simulink model "gm_hybrid_lht"  (R2019b)
settings: Solver=FixedStepDiscrete  StartTime=0.0  StopTime=inf  FixedStep=1/120e6  RelTol=1e-3
undefined symbols (not defined in the file or in its folder): bt, height, nTheta, width
libraries: hdlsllib x672, simulink x614, hdlmdlgenlib x7, dspsrcs4 x1
(part 1 of 18)
settings Model: SimulationMode=accelerator  ExtModeTrigDuration=100  Creator=rgb11127  LastModifiedBy=rgb11127
settings DataIOCC: SaveOutput=off  SaveTime=off  ReturnWorkspaceOutputs=off  StateSaveName=tmp_raccel_xout  SignalLoggingName=tmp_raccel_logsout
settings OptimizationCC: BlockReduction=off  ConditionallyExecuteInputs=off  DefaultParameterBehavior=Inlined  EfficientMapNaN2IntZero=off
settings DebuggingCC: AlgebraicLoopMsg=error  InheritedTsInSrcMsg=none  SingleTaskRateTransMsg=error  ArithmeticOperatorsInVariantConditions=warning
settings HardwareCC: ProdBitPerPointer=32  ProdBitPerSizeT=32  ProdBitPerPtrDiffT=32  ProdLargestAtomicFloat=None  ProdIntDivRoundTo=Undefined  ProdEndianess=Unspecified  ProdWordSize=32  ProdHWDeviceType=ASIC/FPGA->ASIC/FPGA  TargetBitPerPointer=64  TargetBitPerSizeT=64  TargetBitPerPtrDiffT=64  TargetLongLongMode=on  TargetIntDivRoundTo=Zero  TargetEndianess=LittleEndian  TargetWordSize=64  TargetHWDeviceType=Custom Processor->MATLAB Host Computer  ProdEqTarget=off
settings SFSimCC: CustomCodeUndefinedFunction=UseInterfaceOnly
settings RTWCC: SystemTargetFile=raccel.tlc  TemplateMakefile=raccel_default_tmf  RTWVerbose=off  RTWUseSimCustomCode=on
settings CodeAppCC: GenerateComments=off  MaxIdLength=128
settings RaccelTargetCC: GeneratePreprocessorConditionals=Use local settings  MultiInstanceERTCode=off  PreserveStateflowLocalDataDimensions=off  ExtModeMexArgs='', 0, 56287  ENABLE_SLEXEC_SSBRIDGE=1  RTWCAPIParams=on

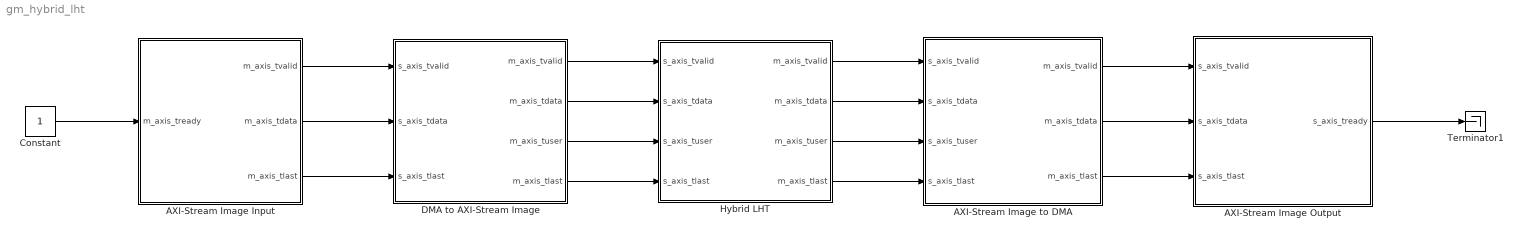
== system gm_hybrid_lht ==
  AXI-Stream Image Input : Subsystem  mask{image=bt.inputImage, clk=1/120e6}
      mask prompts: image "Input Image:"; clk "Clock Rate:"
      mask init:
      | [height, width] = size(image);
      mask DialogControl DescGroupVar Prompt: AXI-Stream Image Input
      mask DialogControl DescTextVar Prompt: This block simulates an AXI-Stream image input for interfacing to a hardware accelerator or IP Core.
      mask DialogControl ParameterGroupVar Prompt: Main
  AXI-Stream Image Output : Subsystem  mask{height=bt.nRho, width=bt.nTheta, clk=1/120e6, d=0}
      mask prompts: height "Image Height:"; width "Image Width:"; clk "Clock Rate:"; d "Frame Capture Number"
      mask DialogControl DescGroupVar Prompt: AXI-Stream Image Output
      mask DialogControl DescTextVar Prompt: Image output using the AXI-Stream interface. Simulates an AXI DMA write channel.
      mask DialogControl ParameterGroupVar Prompt: Main
  AXI-Stream Image to DMA : Subsystem  mask{height=bt.nRho, width=bt.nTheta}
      mask prompts: height "Image Height"; width "Image Width"
      mask DialogControl DescGroupVar Prompt: AXI-Stream Image to DMA
      mask DialogControl DescTextVar Prompt: Converts from the AXI-Stream video standard to AXI-Stream DMA packet.
      mask DialogControl Container2 Prompt: Main
  Constant : Constant  OutDataTypeStr=boolean  SampleTime=-1
  DMA to AXI-Stream Image : Subsystem  mask{height=bt.height, width=bt.width}
      mask prompts: height "Image Height:"; width "Image Width:"
      mask DialogControl DescGroupVar Prompt: DMA to AXI-Stream Image
      mask DialogControl DescTextVar Prompt: Converts an DMA AXI-Stream packet to the AXI-Stream video standard.
      mask DialogControl Container2 Prompt: Main
  Hybrid LHT : Subsystem
  Terminator1 : Terminator
  wires:
  Constant/1 -> AXI-Stream Image Input/1(m_axis_tready)
  AXI-Stream Image Input/1(m_axis_tvalid) -> DMA to AXI-Stream Image/1(s_axis_tvalid)
  AXI-Stream Image Input/2(m_axis_tdata) -> DMA to AXI-Stream Image/2(s_axis_tdata)
  AXI-Stream Image Input/3(m_axis_tlast) -> DMA to AXI-Stream Image/3(s_axis_tlast)
  DMA to AXI-Stream Image/1(m_axis_tvalid) -> Hybrid LHT/1(s_axis_tvalid)
  DMA to AXI-Stream Image/2(m_axis_tdata) -> Hybrid LHT/2(s_axis_tdata)
  DMA to AXI-Stream Image/3(m_axis_tuser) -> Hybrid LHT/3(s_axis_tuser)
  DMA to AXI-Stream Image/4(m_axis_tlast) -> Hybrid LHT/4(s_axis_tlast)
  AXI-Stream Image Output/1(s_axis_tready) -> Terminator1/1
  AXI-Stream Image to DMA/3(m_axis_tlast) -> AXI-Stream Image Output/3(s_axis_tlast)
  AXI-Stream Image to DMA/2(m_axis_tdata) -> AXI-Stream Image Output/2(s_axis_tdata)
  AXI-Stream Image to DMA/1(m_axis_tvalid) -> AXI-Stream Image Output/1(s_axis_tvalid)
  Hybrid LHT/4(m_axis_tlast) -> AXI-Stream Image to DMA/4(s_axis_tlast)
  Hybrid LHT/3(m_axis_tuser) -> AXI-Stream Image to DMA/3(s_axis_tuser)
  Hybrid LHT/2(m_axis_tdata) -> AXI-Stream Image to DMA/2(s_axis_tdata)
  Hybrid LHT/1(m_axis_tvalid) -> AXI-Stream Image to DMA/1(s_axis_tvalid)

== system gm_hybrid_lht/AXI-Stream Image Input ==
  m_axis_tready : Inport
  Compare To Constant : simulink/Logic and Bit Operations/Compare To Constant  relop===  const=height*width-1  OutDataTypeStr=boolean
  Data Type Conversion : DataTypeConversion  OutDataTypeStr=fixdt(0, ceil(log2(max(max(double(image))))), 0)
  HDL Counter : hdlsllib/Sources/HDL Counter  CountType=Count limited  CountInit=0  CountStep=1  CountMax=width*height-1  CountFromType=Initial value  CountFrom=0  CountResetPort=off  CountLoadPort=off  CountEnbPort=on  CountDirPort=off  CountDataType=Unsigned  CountWordLen=ceil(log2(width*height))  CountFracLen=0  CountSampTime=1
      settings: SourceProductName=Simulink
  Master AXI-Stream FIFO : Subsystem  mask{depth=32}
      mask prompts: depth "FIFO Depth:"
      mask DialogControl DescGroupVar Prompt: Master AXI-Stream FIFO
      mask DialogControl DescTextVar Prompt: A custom AXI-Stream FIFO for interfacing to write channel AXI DMAs.
      mask DialogControl ParameterGroupVar Prompt: Main
  Synchronous Image Source : Subsystem
  m_axis_tvalid : Outport
  m_axis_tdata : Outport  Port=2
  m_axis_tlast : Outport  Port=3
  wires:
  Data Type Conversion/1 -> Master AXI-Stream FIFO/2(s_axis_tdata)
  Master AXI-Stream FIFO/2(m_axis_tdata) -> m_axis_tdata/1
  Master AXI-Stream FIFO/3(m_axis_tlast) -> m_axis_tlast/1
  m_axis_tready/1 -> Master AXI-Stream FIFO/4(m_axis_tready)
  Master AXI-Stream FIFO/4(s_axis_tready) -> HDL Counter/1, Master AXI-Stream FIFO/1(s_axis_tvalid), Synchronous Image Source/Enable
  Compare To Constant/1 -> Master AXI-Stream FIFO/3(s_axis_tlast)
  Master AXI-Stream FIFO/1(m_axis_tvalid) -> m_axis_tvalid/1
  HDL Counter/1 -> Compare To Constant/1
  Synchronous Image Source/1(Pixel) -> Data Type Conversion/1

== system gm_hybrid_lht/AXI-Stream Image Output ==
  s_axis_tvalid : Inport
  s_axis_tdata : Inport  Port=2
  s_axis_tlast : Inport  Port=3
  AND1 : Logic  IconShape=distinctive  AllPortsSameDT=off  OutDataTypeStr=boolean
  Compare To Constant4 : simulink/Logic and Bit Operations/Compare To Constant  relop===  const=(height)*width-1  OutDataTypeStr=boolean
  Constant : Constant  OutDataTypeStr=boolean  SampleTime=-1
  Delay2 : Delay  DelayLength=d  ShowEnablePort=on
      settings: InputPortMap=u0,e6
  Pixel to Workspace : Subsystem
  Stop Simulation1 : Stop
  Terminator : Terminator
  Total Samples Counter : hdlsllib/Sources/HDL Counter  CountType=Count limited  CountInit=0  CountStep=1  CountMax=(height)*width-1  CountFromType=Initial value  CountFrom=0  CountResetPort=off  CountLoadPort=off  CountEnbPort=on  CountDirPort=off  CountDataType=Unsigned  CountWordLen=ceil(log2((height)*width+1))  CountFracLen=0  CountSampTime=1
      settings: SourceProductName=Simulink
  s_axis_tready : Outport  VectorParamsAs1DForOutWhenUnconnected=off
  wires:
  Constant/1 -> s_axis_tready/1, AND1/2
  s_axis_tlast/1 -> Terminator/1
  Delay2/1 -> Stop Simulation1/1
  Compare To Constant4/1 -> Delay2/1, Delay2/2
  Total Samples Counter/1 -> Compare To Constant4/1
  AND1/1 -> Pixel to Workspace/Enable, Total Samples Counter/1
  s_axis_tvalid/1 -> AND1/1
  s_axis_tdata/1 -> Pixel to Workspace/1(Pixel In)

== system gm_hybrid_lht/AXI-Stream Image to DMA ==
  s_axis_tvalid : Inport
  s_axis_tdata : Inport  Port=2
  s_axis_tuser : Inport  Port=3
  s_axis_tlast : Inport  Port=4
  AND : Logic  IconShape=distinctive  AllPortsSameDT=off  OutDataTypeStr=boolean
  Compare To Constant : simulink/Logic and Bit Operations/Compare To Constant  relop===  const=height*width-1  OutDataTypeStr=boolean
  Data Type Conversion : DataTypeConversion  OutDataTypeStr=uint32
  Output Counter : hdlsllib/Sources/HDL Counter  CountType=Count limited  CountInit=0  CountStep=1  CountMax=height*width-1  CountFromType=Initial value  CountFrom=0  CountResetPort=off  CountLoadPort=off  CountEnbPort=on  CountDirPort=off  CountDataType=Unsigned  CountWordLen=ceil(log2(height*width))  CountFracLen=0  CountSampTime=1
      settings: SourceProductName=Simulink
  Terminator : Terminator
  Terminator1 : Terminator
  m_axis_tvalid : Outport
  m_axis_tdata : Outport  Port=2
  m_axis_tlast : Outport  Port=3
  wires:
  Data Type Conversion/1 -> m_axis_tdata/1
  s_axis_tdata/1 -> Data Type Conversion/1
  s_axis_tvalid/1 -> AND/2, m_axis_tvalid/1, Output Counter/1
  s_axis_tlast/1 -> Terminator/1
  s_axis_tuser/1 -> Terminator1/1
  Output Counter/1 -> Compare To Constant/1
  Compare To Constant/1 -> AND/1
  AND/1 -> m_axis_tlast/1

== system gm_hybrid_lht/DMA to AXI-Stream Image ==
  s_axis_tvalid : Inport
  s_axis_tdata : Inport  Port=2
  s_axis_tlast : Inport  Port=3
  AND : Logic  IconShape=distinctive  AllPortsSameDT=off  OutDataTypeStr=boolean
  AND1 : Logic  IconShape=distinctive  AllPortsSameDT=off  OutDataTypeStr=boolean
  AND2 : Logic  IconShape=distinctive  AllPortsSameDT=off  OutDataTypeStr=boolean
  Compare To Constant : simulink/Logic and Bit Operations/Compare To Constant  relop===  const=width-1  OutDataTypeStr=boolean
  Compare To Zero : simulink/Logic and Bit Operations/Compare To Zero  relop===  OutDataTypeStr=boolean
  Compare To Zero1 : simulink/Logic and Bit Operations/Compare To Zero  relop===  OutDataTypeStr=boolean
  Terminator : Terminator
  X Counter : hdlsllib/Sources/HDL Counter  CountType=Count limited  CountInit=0  CountStep=1  CountMax=width-1  CountFromType=Initial value  CountFrom=0  CountResetPort=off  CountLoadPort=off  CountEnbPort=on  CountDirPort=off  CountDataType=Unsigned  CountWordLen=ceil(log2(width))  CountFracLen=0  CountSampTime=1
      settings: SourceProductName=Simulink
  Y Counter : hdlsllib/Sources/HDL Counter  CountType=Count limited  CountInit=0  CountStep=1  CountMax=height-1  CountFromType=Initial value  CountFrom=0  CountResetPort=off  CountLoadPort=off  CountEnbPort=on  CountDirPort=off  CountDataType=Unsigned  CountWordLen=ceil(log2(height))  CountFracLen=0  CountSampTime=1
      settings: SourceProductName=Simulink
  m_axis_tvalid : Outport
  m_axis_tdata : Outport  Port=2
  m_axis_tuser : Outport  Port=3
  m_axis_tlast : Outport  Port=4
  wires:
  AND2/1 -> m_axis_tlast/1
  Compare To Constant/1 -> Y Counter/1, AND2/2
  AND1/1 -> m_axis_tuser/1
  AND/1 -> AND1/2
  s_axis_tlast/1 -> Terminator/1
  Compare To Zero/1 -> AND/2
  Compare To Zero1/1 -> AND/1
  Y Counter/1 -> Compare To Zero/1
  X Counter/1 -> Compare To Constant/1, Compare To Zero1/1
  s_axis_tvalid/1 -> m_axis_tvalid/1, AND1/1, AND2/1, X Counter/1
  s_axis_tdata/1 -> m_axis_tdata/1

== system gm_hybrid_lht/Hybrid LHT ==
  s_axis_tvalid : Inport  OutDataTypeStr=boolean  PortDimensions=1  SampleTime=8.33333333333333e-09
  s_axis_tdata : Inport  Port=2  OutDataTypeStr=fixdt(0, 9, 0)  PortDimensions=1  SampleTime=8.33333333333333e-09
  s_axis_tuser : Inport  Port=3  OutDataTypeStr=boolean  PortDimensions=1  SampleTime=8.33333333333333e-09
  s_axis_tlast : Inport  Port=4  OutDataTypeStr=boolean  PortDimensions=1  SampleTime=8.33333333333333e-09
  Hybrid LHT Accumulator : Subsystem  mask{height=double(1080), width=double(1920), theta=reshape(double([0 1 2 3 4 5 6 7 8 9 10 11 12 13 14 15 16 17 18 19 20 21 22 23 24 25 26 27 28 29 30 31 32 33 34 35 36 37 38 39 40 41 42 43 44 45 46 47 48 49 50 51 52 53 54 55 56 57 58 59 60 61 62 63 64 65 66 67 68 69 70 71 72 73 74 75 76 77 78 79 80 81 82 83 84 85 86 87 88 89 90 91 92 93 94 95 96 97 98 99 100 101 102 103 104 105 106 107 108 109 110 111 112 113 114 115 116 117 118 119 120 121 122 123 124 125 126 127 128 129 130 131 132 133 134 135 136 137 138 139 140 141 142 143 144 145 146 147 148 149 150 151 152 153 154 155 156 157 158 159 160 161 162 163 164 165 166 167 168 169 170 171 172 173 174 175 176 177 178 179]).', [1  180])}
      mask prompts: height "Image Height:"; width "Image Width:"; theta "Orientations:"
      mask init:
      | maxRho = ceil(sqrt((height/2)^2+(width/2)^2));
      | nRho = maxRho*2;
      | [~, nTheta] = size(theta);
      | 
      | voteWL = ceil(log2(2*maxRho));
  Hybrid LHT Kernel : Subsystem  mask{height=double(1080), width=double(1920), theta=reshape(double([0 1 2 3 4 5 6 7 8 9 10 11 12 13 14 15 16 17 18 19 20 21 22 23 24 25 26 27 28 29 30 31 32 33 34 35 36 37 38 39 40 41 42 43 44 45 46 47 48 49 50 51 52 53 54 55 56 57 58 59 60 61 62 63 64 65 66 67 68 69 70 71 72 73 74 75 76 77 78 79 80 81 82 83 84 85 86 87 88 89 90 91 92 93 94 95 96 97 98 99 100 101 102 103 104 105 106 107 108 109 110 111 112 113 114 115 116 117 118 119 120 121 122 123 124 125 126 127 128 129 130 131 132 133 134 135 136 137 138 139 140 141 142 143 144 145 146 147 148 149 150 151 152 153 154 155 156 157 158 159 160 161 162 163 164 165 166 167 168 169 170 171 172 173 174 175 176 177 178 179]).', [1  180])}
      mask prompts: height "Image Height:"; width "Image Width:"; theta "Orientations:"
      mask init:
      | % Get number of orientations to operate across
      | [~, nTheta] = size(theta);
      | 
      | % Get discretisation step of theta
      | if nTheta > 1
      |     dTheta = theta(end) - theta(end-1);
      | else
      |     dTheta = 1;
      | end
      | 
      | % Get the maximum magnitude of displacement
      | maxRho = ceil(sqrt((height/2)^2+(width/2)^2));
      | 
      | % Get the number of bits required to vote correctly
      | voteWL = ceil(log2(maxRho*2));
      | 
      | % Get the number of division possible
      | if nTheta < floor(36/voteWL)
      |     L = nTheta;
      | else
      |     L = floor(36/voteWL);
      | end
      | 
      | % Set lambda, the number of orientations to operate across per gradient
      | % orientation given
      | lambda = floor(nTheta/(2*L));
      | 
      | % Determine if the number of orientations is odd. This will prevent over
      | % use of the parameter space.
      | if lambda == 0
      |     subflag = 0;
      | else
      |     subflag = ~mod(nTheta/(L), 2);
      | end
      | 
      | % Get the limits so that we can determine the number of bits to shift
      | % the votes
      | U = floor(nTheta/L):floor(nTheta/L):nTheta;
      | D = 0:floor(nTheta/L):nTheta-1;
  delayMatch : Delay  DelayLength=double(2)  InitialCondition=0  SampleTime=8.33333333333333e-09
  delayMatch1 : Delay  DelayLength=double(2)  InitialCondition=0  SampleTime=8.33333333333333e-09
  m_axis_tvalid : Outport
  m_axis_tdata : Outport  Port=2
  m_axis_tuser : Outport  Port=3
  m_axis_tlast : Outport  Port=4
  wires:
  s_axis_tvalid/1 -> Hybrid LHT Kernel/1(s_axis_tvalid)
  s_axis_tdata/1 -> Hybrid LHT Kernel/2(s_axis_tdata)
  s_axis_tuser/1 -> Hybrid LHT Kernel/3(s_axis_tuser)
  s_axis_tlast/1 -> Hybrid LHT Kernel/4(s_axis_tlast)
  delayMatch/1 -> m_axis_tvalid/1
  Hybrid LHT Accumulator/2(m_axis_tdata) -> m_axis_tdata/1
  Hybrid LHT Accumulator/3(m_axis_tuser) -> m_axis_tuser/1
  delayMatch1/1 -> m_axis_tlast/1
  Hybrid LHT Kernel/1(m_axis_tvalid) -> Hybrid LHT Accumulator/1(s_axis_tvalid)
  Hybrid LHT Kernel/2(m_axis_tuser) -> Hybrid LHT Accumulator/2(s_axis_tuser)
  Hybrid LHT Kernel/3(m_axis_tlast) -> Hybrid LHT Accumulator/3(s_axis_tlast)
  Hybrid LHT Kernel/4(hough_param) -> Hybrid LHT Accumulator/4(hough_param)
  Hybrid LHT Kernel/5(edge) -> Hybrid LHT Accumulator/5(edge)
  Hybrid LHT Kernel/6(shift) -> Hybrid LHT Accumulator/6(shift)
  Hybrid LHT Accumulator/1(m_axis_tvalid) -> delayMatch/1
  Hybrid LHT Accumulator/4(m_axis_tlast) -> delayMatch1/1

== system gm_hybrid_lht/AXI-Stream Image Input/Master AXI-Stream FIFO ==
  s_axis_tvalid : Inport
  s_axis_tdata : Inport  Port=2
  s_axis_tlast : Inport  Port=3
  m_axis_tready : Inport  Port=4
  AND : Logic  IconShape=distinctive  AllPortsSameDT=off  OutDataTypeStr=boolean
  "Compare To Constant " : simulink/Logic and Bit Operations/Compare To Constant  relop=>=  const=floor(depth/2)  OutDataTypeStr=boolean
  Delay : Delay  DelayLength=1
  HDL FIFO TDATA : hdlsllib/HDL RAMs/HDL FIFO  fifo_size=depth  mode=Classic  ratio=1  push_msg=Error  pop_msg=Error  show_empty=on  show_full=off  show_num=on  LabelModeActiveChoice_Mode=Classic
      settings: SourceProductName=Simulink  SourceProductBaseCode=SL
  HDL FIFO TLAST : hdlsllib/HDL RAMs/HDL FIFO  fifo_size=depth  mode=Classic  ratio=1  push_msg=Error  pop_msg=Error  show_empty=off  show_full=off  show_num=off  LabelModeActiveChoice_Mode=Classic
      settings: SourceProductName=Simulink  SourceProductBaseCode=SL
  NOT : Logic  Operator=NOT  IconShape=distinctive  AllPortsSameDT=off  OutDataTypeStr=boolean
  NOT1 : Logic  Operator=NOT  IconShape=distinctive  AllPortsSameDT=off  OutDataTypeStr=boolean
  m_axis_tvalid : Outport  VectorParamsAs1DForOutWhenUnconnected=off
  m_axis_tdata : Outport  Port=2  VectorParamsAs1DForOutWhenUnconnected=off
  m_axis_tlast : Outport  Port=3  VectorParamsAs1DForOutWhenUnconnected=off
  s_axis_tready : Outport  Port=4
  wires:
  Delay/1 -> m_axis_tvalid/1
  s_axis_tvalid/1 -> HDL FIFO TDATA/2, HDL FIFO TLAST/2
  s_axis_tdata/1 -> HDL FIFO TDATA/1
  s_axis_tlast/1 -> HDL FIFO TLAST/1
  "Compare To Constant "/1 -> NOT1/1
  NOT1/1 -> s_axis_tready/1
  HDL FIFO TDATA/3 -> "Compare To Constant "/1
  m_axis_tready/1 -> AND/1
  NOT/1 -> AND/2, Delay/1
  AND/1 -> HDL FIFO TDATA/3, HDL FIFO TLAST/3
  HDL FIFO TDATA/2 -> NOT/1
  HDL FIFO TLAST/1 -> m_axis_tlast/1
  HDL FIFO TDATA/1 -> m_axis_tdata/1

== system gm_hybrid_lht/AXI-Stream Image Input/Synchronous Image Source ==
  Enable : EnablePort
  Signal From Workspace : dspsrcs4/Signal From Workspace  X=reshape((double(image))', [height*width, 1])  Ts=clk  nsamps=1  OutputAfterFinalValue=Cyclic repetition  ignoreOrWarnInputAndFrameLengths=off  OutputFrames=off
  Pixel : Outport
  wires:
  Signal From Workspace/1 -> Pixel/1

== system gm_hybrid_lht/AXI-Stream Image Output/Pixel to Workspace ==
  Pixel In : Inport
  Enable : EnablePort
  To Workspace : ToWorkspace  VariableName=simout  SampleTime=-1
      settings: MaxDataPoints=height*width  Save2DSignal=2-D array (concatenate along first dimension)
  wires:
  Pixel In/1 -> To Workspace/1

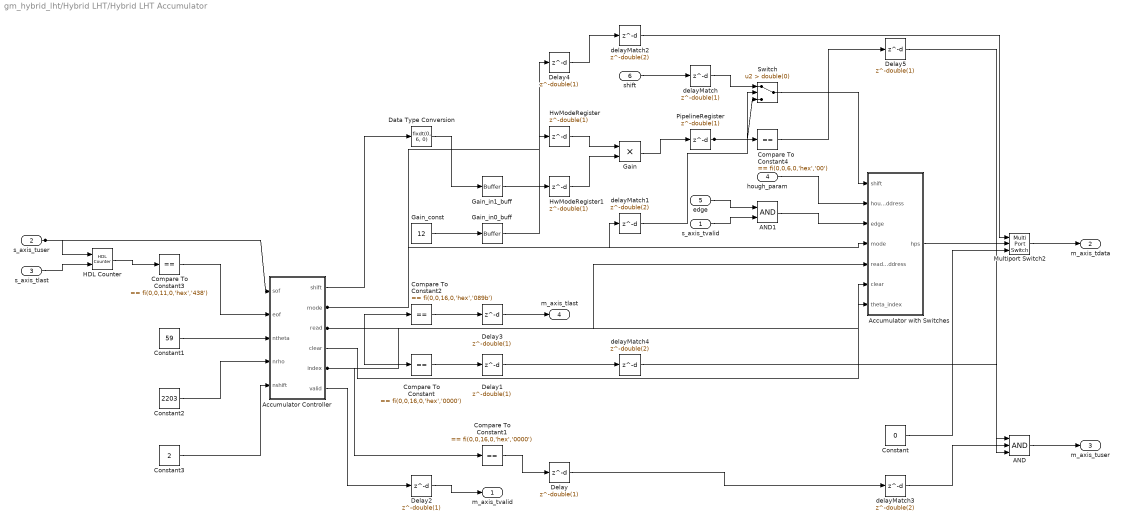
== system gm_hybrid_lht/Hybrid LHT/Hybrid LHT Accumulator ==
  s_axis_tvalid : Inport  OutDataTypeStr=boolean  PortDimensions=1  SampleTime=8.33333333333333e-09
  s_axis_tuser : Inport  Port=2  OutDataTypeStr=boolean  PortDimensions=1  SampleTime=8.33333333333333e-09
  s_axis_tlast : Inport  Port=3  OutDataTypeStr=boolean  PortDimensions=1  SampleTime=8.33333333333333e-09
  hough_param : Inport  Port=4  OutDataTypeStr=fixdt(0, 12, 0)  PortDimensions=[1 60]  SampleTime=8.33333333333333e-09
  edge : Inport  Port=5  OutDataTypeStr=fixdt(0, 1, 0)  PortDimensions=1  SampleTime=8.33333333333333e-09
  shift : Inport  Port=6  OutDataTypeStr=fixdt(0, 6, 0)  PortDimensions=[1 60]  SampleTime=8.33333333333333e-09
  AND : Logic  Inputs=3  AllPortsSameDT=off  OutDataTypeStr=boolean  SampleTime=8.33333333333333e-09
  AND1 : Logic  AllPortsSameDT=off  OutDataTypeStr=boolean  SampleTime=8.33333333333333e-09
  Accumulator Controller : Subsystem
  Accumulator with Switches : Subsystem
  Compare To Constant : simulink/Logic and Bit Operations/Compare To Constant  relop===  const=fi(0,0,16,0,'hex','0000')  OutDataTypeStr=boolean
  Compare To Constant1 : simulink/Logic and Bit Operations/Compare To Constant  relop===  const=fi(0,0,16,0,'hex','0000')  OutDataTypeStr=boolean
  Compare To Constant2 : simulink/Logic and Bit Operations/Compare To Constant  relop===  const=fi(0,0,16,0,'hex','089b')  OutDataTypeStr=boolean
  Compare To Constant3 : simulink/Logic and Bit Operations/Compare To Constant  relop===  const=fi(0,0,11,0,'hex','438')  OutDataTypeStr=boolean
  Compare To Constant4 : simulink/Logic and Bit Operations/Compare To Constant  relop===  const=fi(0,0,6,0,'hex','00')  OutDataTypeStr=boolean
  Constant : Constant  Value=0  OutDataTypeStr=fixdt(0, 12, 0)  SampleTime=-1
  Constant1 : Constant  Value=59  OutDataTypeStr=uint16  SampleTime=-1
  Constant2 : Constant  Value=2203  OutDataTypeStr=uint16  SampleTime=-1
  Constant3 : Constant  Value=2  OutDataTypeStr=fixdt(0, 3, 0)  SampleTime=-1
  Data Type Conversion : DataTypeConversion  OutDataTypeStr=fixdt(0, 6, 0)  SampleTime=8.33333333333333e-09
  Delay{,1..5} (6 alike) : Delay  DelayLength=double(1)  InitialCondition=0  SampleTime=8.33333333333333e-09
  Gain : Product  Inputs=**  OutDataTypeStr=fixdt(0, 6, 0)  SampleTime=8.33333333333333e-09
  Gain_const : Constant  Value=12  OutDataTypeStr=fixdt(0, 6, 2)  SampleTime=-1
  Gain_in0_buff : hdlmdlgenlib/Buffer
      settings: SourceProductName=Simulink  SourceProductBaseCode=SL
  Gain_in1_buff : hdlmdlgenlib/Buffer
      settings: SourceProductName=Simulink  SourceProductBaseCode=SL
  HDL Counter : hdlsllib/Sources/HDL Counter  CountType=Count limited  CountInit=double(0)  CountStep=double(1)  CountMax=double(1080)  CountFromType=Initial value  CountFrom=double(0)  CountResetPort=on  CountLoadPort=off  CountEnbPort=on  CountDirPort=off  CountDataType=Unsigned  CountWordLen=11  CountFracLen=0  CountSampTime=8.33333333333333e-09
      settings: SourceProductName=Simulink
  HwModeRegister : Delay  DelayLength=double(1)  InitialCondition=0  SampleTime=8.33333333333333e-09
  HwModeRegister1 : Delay  DelayLength=double(1)  InitialCondition=0  SampleTime=8.33333333333333e-09
  Multiport Switch2 : MultiPortSwitch  DataPortOrder=Zero-based contiguous  Inputs=2  DiagnosticForDefault=None  zeroidx=on  OutDataTypeStr=fixdt(0, 12, 0)  SampleTime=8.33333333333333e-09
  PipelineRegister : Delay  DelayLength=double(1)  InitialCondition=0  SampleTime=8.33333333333333e-09
  Switch : Switch  Criteria=u2 > Threshold  Threshold=double(0)  OutDataTypeStr=fixdt(0, 6, 0)  SampleTime=8.33333333333333e-09
  delayMatch : Delay  DelayLength=double(1)  InitialCondition=0  SampleTime=8.33333333333333e-09
  delayMatch{1..4} (4 alike) : Delay  DelayLength=double(2)  InitialCondition=0  SampleTime=8.33333333333333e-09
  m_axis_tvalid : Outport
  m_axis_tdata : Outport  Port=2
  m_axis_tuser : Outport  Port=3
  m_axis_tlast : Outport  Port=4
  wires:
  delayMatch/1 -> Switch/1
  AND/1 -> m_axis_tuser/1
  AND1/1 -> Accumulator with Switches/3(edge)
  Accumulator Controller/1(shift) -> Data Type Conversion/1
  delayMatch1/1 -> Switch/2
  Accumulator Controller/3(read) -> Compare To Constant2/1, Compare To Constant/1, Accumulator with Switches/5(read_address)
  Accumulator Controller/4(clear) -> Accumulator with Switches/6(clear)
  Accumulator Controller/5(index) -> Compare To Constant1/1, Accumulator with Switches/7(theta_index)
  Accumulator Controller/6(valid) -> Delay2/1
  Accumulator with Switches/1(hps) -> Multiport Switch2/2
  Compare To Constant/1 -> Delay1/1
  Compare To Constant1/1 -> Delay/1
  Compare To Constant2/1 -> Delay3/1
  Compare To Constant3/1 -> Accumulator Controller/2(eof)
  Compare To Constant4/1 -> Delay5/1
  Constant/1 -> Multiport Switch2/3
  Constant1/1 -> Accumulator Controller/3(ntheta)
  Constant2/1 -> Accumulator Controller/4(nrho)
  Constant3/1 -> Accumulator Controller/5(nshift)
  Data Type Conversion/1 -> Gain_in1_buff/1
  delayMatch3/1 -> AND/2
  delayMatch4/1 -> AND/3
  Delay2/1 -> m_axis_tvalid/1
  Delay3/1 -> m_axis_tlast/1
  delayMatch2/1 -> Multiport Switch2/1
  Delay5/1 -> AND/1
  PipelineRegister/1 -> Switch/3, Compare To Constant4/1
  HDL Counter/1 -> Compare To Constant3/1
  Multiport Switch2/1 -> m_axis_tdata/1
  Switch/1 -> Accumulator with Switches/1(shift)
  Gain_const/1 -> Gain_in0_buff/1
  s_axis_tvalid/1 -> AND1/2
  s_axis_tuser/1 -> HDL Counter/1, Accumulator Controller/1(sof)
  s_axis_tlast/1 -> HDL Counter/2
  hough_param/1 -> Accumulator with Switches/2(hough_address)
  edge/1 -> AND1/1
  shift/1 -> delayMatch/1
  Accumulator Controller/2(mode) -> delayMatch1/1, Delay4/1, Accumulator with Switches/4(mode)
  Delay4/1 -> delayMatch2/1
  Delay/1 -> delayMatch3/1
  Delay1/1 -> delayMatch4/1
  Gain/1 -> PipelineRegister/1
  HwModeRegister/1 -> Gain/1
  HwModeRegister1/1 -> Gain/2
  Gain_in0_buff/1 -> HwModeRegister/1
  Gain_in1_buff/1 -> HwModeRegister1/1

== system gm_hybrid_lht/Hybrid LHT/Hybrid LHT Kernel ==
  s_axis_tvalid : Inport  OutDataTypeStr=boolean  PortDimensions=1  SampleTime=8.33333333333333e-09
  s_axis_tdata : Inport  Port=2  OutDataTypeStr=fixdt(0, 9, 0)  PortDimensions=1  SampleTime=8.33333333333333e-09
  s_axis_tuser : Inport  Port=3  OutDataTypeStr=boolean  PortDimensions=1  SampleTime=8.33333333333333e-09
  s_axis_tlast : Inport  Port=4  OutDataTypeStr=boolean  PortDimensions=1  SampleTime=8.33333333333333e-09
  AND : Logic  AllPortsSameDT=off  OutDataTypeStr=boolean  SampleTime=8.33333333333333e-09
  Edge Slice : hdlsllib/Logic and Bit Operations/Bit Slice  lidx=double(8)  ridx=double(8)
      settings: SourceProductName=Simulink  SourceProductBaseCode=SL
  Extract Active Votes : Subsystem
  Gradient Kernel System : Subsystem
  Selector1 : Selector  NumberOfDimensions=2  IndexMode=Zero-based  SampleTime=8.33333333333333e-09  IndexOptions=Index vector (dialog),Index vector (port)  Indices=double(0),double(1)  OutputSizes=double(1),double(1)
  Selector6 : Selector  NumberOfDimensions=2  IndexMode=Zero-based  SampleTime=8.33333333333333e-09  IndexOptions=Index vector (dialog),Index vector (port)  Indices=double(0),double(1)  OutputSizes=double(1),double(1)
  Theta Slice : hdlsllib/Logic and Bit Operations/Bit Slice  lidx=double(7)  ridx=double(0)
      settings: SourceProductName=Simulink  SourceProductBaseCode=SL
  X Counter : hdlsllib/Sources/HDL Counter  CountType=Count limited  CountInit=double(-960)  CountStep=double(1)  CountMax=double(959)  CountFromType=Initial value  CountFrom=double(-960)  CountResetPort=off  CountLoadPort=off  CountEnbPort=on  CountDirPort=off  CountDataType=Signed  CountWordLen=11  CountFracLen=0  CountSampTime=8.33333333333333e-09
      settings: SourceProductName=Simulink
  Y Counter : hdlsllib/Sources/HDL Counter  CountType=Count limited  CountInit=double(-540)  CountStep=double(1)  CountMax=double(539)  CountFromType=Initial value  CountFrom=double(-540)  CountResetPort=off  CountLoadPort=off  CountEnbPort=on  CountDirPort=off  CountDataType=Signed  CountWordLen=11  CountFracLen=0  CountSampTime=8.33333333333333e-09
      settings: SourceProductName=Simulink
  delayMatch : Delay  DelayLength=double(1)  InitialCondition=0  SampleTime=8.33333333333333e-09
  m_axis_tvalid : Outport
  m_axis_tuser : Outport  Port=2
  m_axis_tlast : Outport  Port=3
  hough_param : Outport  Port=4
  edge : Outport  Port=5
  shift : Outport  Port=6
  wires:
  AND/1 -> Y Counter/1
  Edge Slice/1 -> Gradient Kernel System/1(Edge)
  delayMatch/1 -> Selector6/2
  Gradient Kernel System/1(vEdge) -> edge/1
  Gradient Kernel System/2(Rho) -> Selector6/1
  Gradient Kernel System/3(Shift) -> Selector1/1
  Selector1/1 -> shift/1
  Selector6/1 -> hough_param/1
  Theta Slice/1 -> Gradient Kernel System/4(Theta), Extract Active Votes/1(Theta)
  X Counter/1 -> Gradient Kernel System/2(X)
  Y Counter/1 -> Gradient Kernel System/3(Y)
  s_axis_tvalid/1 -> AND/1, X Counter/1, m_axis_tvalid/1
  s_axis_tdata/1 -> Theta Slice/1, Edge Slice/1
  s_axis_tuser/1 -> m_axis_tuser/1
  s_axis_tlast/1 -> AND/2, m_axis_tlast/1
  Extract Active Votes/1(Index) -> delayMatch/1, Selector1/2

== system gm_hybrid_lht/Hybrid LHT/Hybrid LHT Accumulator/Accumulator Controller ==
  sof : Inport  OutDataTypeStr=boolean  PortDimensions=1  SampleTime=8.33333333333333e-09
  eof : Inport  Port=2  OutDataTypeStr=boolean  PortDimensions=1  SampleTime=8.33333333333333e-09
  ntheta : Inport  Port=3  OutDataTypeStr=uint16  PortDimensions=1  SampleTime=8.33333333333333e-09
  nrho : Inport  Port=4  OutDataTypeStr=uint16  PortDimensions=1  SampleTime=8.33333333333333e-09
  nshift : Inport  Port=5  OutDataTypeStr=fixdt(0, 3, 0)  PortDimensions=1  SampleTime=8.33333333333333e-09
  Accumulator Controller : MATLAB Function  TreatAsAtomicUnit=on
  shift : Outport
  mode : Outport  Port=2
  read : Outport  Port=3
  clear : Outport  Port=4
  index : Outport  Port=5
  valid : Outport  Port=6
  wires:
  Accumulator Controller/1(shift) -> shift/1
  Accumulator Controller/2(mode) -> mode/1
  Accumulator Controller/3(read) -> read/1
  Accumulator Controller/4(clear) -> clear/1
  Accumulator Controller/5(index) -> index/1
  Accumulator Controller/6(valid) -> valid/1
  sof/1 -> Accumulator Controller/1(sof)
  eof/1 -> Accumulator Controller/2(eof)
  ntheta/1 -> Accumulator Controller/3(ntheta)
  nrho/1 -> Accumulator Controller/4(nrho)
  nshift/1 -> Accumulator Controller/5(nshift)

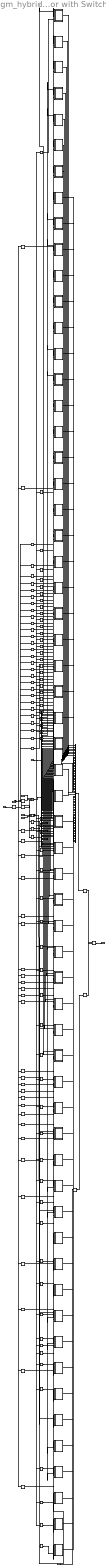
== system gm_hybrid_lht/Hybrid LHT/Hybrid LHT Accumulator/Accumulator with Switches ==
  shift : Inport  OutDataTypeStr=fixdt(0, 6, 0)  PortDimensions=[1 60]  SampleTime=8.33333333333333e-09
  hough_address : Inport  Port=2  OutDataTypeStr=fixdt(0, 12, 0)  PortDimensions=[1 60]  SampleTime=8.33333333333333e-09
  edge : Inport  Port=3  OutDataTypeStr=boolean  PortDimensions=1  SampleTime=8.33333333333333e-09
  mode : Inport  Port=4  OutDataTypeStr=boolean  PortDimensions=1  SampleTime=8.33333333333333e-09
  read_address : Inport  Port=5  OutDataTypeStr=uint16  PortDimensions=1  SampleTime=8.33333333333333e-09
  clear : Inport  Port=6  OutDataTypeStr=boolean  PortDimensions=1  SampleTime=8.33333333333333e-09
  theta_index : Inport  Port=7  OutDataTypeStr=uint16  PortDimensions=1  SampleTime=8.33333333333333e-09
  Accumulator_instance1 : Subsystem
  Accumulator_instance10 : Subsystem
  Accumulator_instance11 : Subsystem
  Accumulator_instance12 : Subsystem
  Accumulator_instance13 : Subsystem
  Accumulator_instance14 : Subsystem
  Accumulator_instance15 : Subsystem
  Accumulator_instance16 : Subsystem
  Accumulator_instance17 : Subsystem
  Accumulator_instance18 : Subsystem
  Accumulator_instance19 : Subsystem
  Accumulator_instance2 : Subsystem
  Accumulator_instance20 : Subsystem
  Accumulator_instance21 : Subsystem
  Accumulator_instance22 : Subsystem
  Accumulator_instance23 : Subsystem
  Accumulator_instance24 : Subsystem
  Accumulator_instance25 : Subsystem
  Accumulator_instance26 : Subsystem
  Accumulator_instance27 : Subsystem
  Accumulator_instance28 : Subsystem
  Accumulator_instance29 : Subsystem
  Accumulator_instance3 : Subsystem
  Accumulator_instance30 : Subsystem
  Accumulator_instance31 : Subsystem
  Accumulator_instance32 : Subsystem
  Accumulator_instance33 : Subsystem
  Accumulator_instance34 : Subsystem
  Accumulator_instance35 : Subsystem
  Accumulator_instance36 : Subsystem
  Accumulator_instance37 : Subsystem
  Accumulator_instance38 : Subsystem
  Accumulator_instance39 : Subsystem
  Accumulator_instance4 : Subsystem
  Accumulator_instance40 : Subsystem
  Accumulator_instance41 : Subsystem
  Accumulator_instance42 : Subsystem
  Accumulator_instance43 : Subsystem
  Accumulator_instance44 : Subsystem
  Accumulator_instance45 : Subsystem
  Accumulator_instance46 : Subsystem
  Accumulator_instance47 : Subsystem
  Accumulator_instance48 : Subsystem
  Accumulator_instance49 : Subsystem
  Accumulator_instance5 : Subsystem
  Accumulator_instance50 : Subsystem
  Accumulator_instance51 : Subsystem
  Accumulator_instance52 : Subsystem
  Accumulator_instance53 : Subsystem
  Accumulator_instance54 : Subsystem
  Accumulator_instance55 : Subsystem
  Accumulator_instance56 : Subsystem
  Accumulator_instance57 : Subsystem
  Accumulator_instance58 : Subsystem
  Accumulator_instance59 : Subsystem
  Accumulator_instance6 : Subsystem
  Accumulator_instance60 : Subsystem
  Accumulator_instance7 : Subsystem
  Accumulator_instance8 : Subsystem
  Accumulator_instance9 : Subsystem
  Data Type Conversion : DataTypeConversion  OutDataTypeStr=fixdt(0, 12, 0)  SampleTime=8.33333333333333e-09
  Delay : Delay  DelayLength=double(1)  InitialCondition=0  SampleTime=8.33333333333333e-09
  Multiport Switch1 : MultiPortSwitch  DataPortOrder=Zero-based contiguous  Inputs=2  DiagnosticForDefault=None  zeroidx=on  SampleTime=8.33333333333333e-09
  Selector : Selector  NumberOfDimensions=2  IndexMode=Zero-based  SampleTime=8.33333333333333e-09  IndexOptions=Index vector (dialog),Index vector (port)  Indices=double(0),double(0)  OutputSizes=double(1),double(1)
  Switch : Switch  Criteria=u2 > Threshold  Threshold=double(0)  OutDataTypeStr=fixdt(0, 12, 0)  SampleTime=8.33333333333333e-09
  delayMatch{,1..122} (123 alike) : Delay  DelayLength=double(2)  InitialCondition=0  SampleTime=8.33333333333333e-09
  t : Demux  Outputs=60
  t1 : Demux  Outputs=60
  t2 : Concatenate  NumInputs=60
  t3 : Reshape  OutputDimensionality=Row vector (2-D)
  hps : Outport
  wires:
  delayMatch/1 -> Switch/2
  t3/1 -> Selector/1
  delayMatch1/1 -> Switch/3
  delayMatch122/1 -> Selector/2
  delayMatch3/1 -> Accumulator_instance1/4(edge)
  Selector/1 -> hps/1
  Switch/1 -> t1/1
  t/1 -> Accumulator_instance1/1(shift)
  t/2 -> Accumulator_instance2/1(shift)
  t/3 -> Accumulator_instance3/1(shift)
  t/4 -> Accumulator_instance4/1(shift)
  t/5 -> Accumulator_instance5/1(shift)
  t/6 -> Accumulator_instance6/1(shift)
  t/7 -> Accumulator_instance7/1(shift)
  t/8 -> Accumulator_instance8/1(shift)
  t/9 -> Accumulator_instance9/1(shift)
  t/10 -> Accumulator_instance10/1(shift)
  t/11 -> Accumulator_instance11/1(shift)
  t/12 -> Accumulator_instance12/1(shift)
  t/13 -> Accumulator_instance13/1(shift)
  t/14 -> Accumulator_instance14/1(shift)
  t/15 -> Accumulator_instance15/1(shift)
  t/16 -> Accumulator_instance16/1(shift)
  t/17 -> Accumulator_instance17/1(shift)
  t/18 -> Accumulator_instance18/1(shift)
  t/19 -> Accumulator_instance19/1(shift)
  t/20 -> Accumulator_instance20/1(shift)
  t/21 -> Accumulator_instance21/1(shift)
  t/22 -> Accumulator_instance22/1(shift)
  t/23 -> Accumulator_instance23/1(shift)
  t/24 -> Accumulator_instance24/1(shift)
  t/25 -> Accumulator_instance25/1(shift)
  t/26 -> Accumulator_instance26/1(shift)
  t/27 -> Accumulator_instance27/1(shift)
  t/28 -> Accumulator_instance28/1(shift)
  t/29 -> Accumulator_instance29/1(shift)
  t/30 -> Accumulator_instance30/1(shift)
  t/31 -> Accumulator_instance31/1(shift)
  t/32 -> Accumulator_instance32/1(shift)
  t/33 -> Accumulator_instance33/1(shift)
  t/34 -> Accumulator_instance34/1(shift)
  t/35 -> Accumulator_instance35/1(shift)
  t/36 -> Accumulator_instance36/1(shift)
  t/37 -> Accumulator_instance37/1(shift)
  t/38 -> Accumulator_instance38/1(shift)
  t/39 -> Accumulator_instance39/1(shift)
  t/40 -> Accumulator_instance40/1(shift)
  t/41 -> Accumulator_instance41/1(shift)
  t/42 -> Accumulator_instance42/1(shift)
  t/43 -> Accumulator_instance43/1(shift)
  t/44 -> Accumulator_instance44/1(shift)
  t/45 -> Accumulator_instance45/1(shift)
  t/46 -> Accumulator_instance46/1(shift)
  t/47 -> Accumulator_instance47/1(shift)
  t/48 -> Accumulator_instance48/1(shift)
  t/49 -> Accumulator_instance49/1(shift)
  t/50 -> Accumulator_instance50/1(shift)
  t/51 -> Accumulator_instance51/1(shift)
  t/52 -> Accumulator_instance52/1(shift)
  t/53 -> Accumulator_instance53/1(shift)
  t/54 -> Accumulator_instance54/1(shift)
  t/55 -> Accumulator_instance55/1(shift)
  t/56 -> Accumulator_instance56/1(shift)
  t/57 -> Accumulator_instance57/1(shift)
  t/58 -> Accumulator_instance58/1(shift)
  t/59 -> Accumulator_instance59/1(shift)
  t/60 -> Accumulator_instance60/1(shift)
  t1/1 -> Accumulator_instance1/3(address)
  t1/2 -> Accumulator_instance2/3(address)
  t1/3 -> Accumulator_instance3/3(address)
  t1/4 -> Accumulator_instance4/3(address)
  t1/5 -> Accumulator_instance5/3(address)
  t1/6 -> Accumulator_instance6/3(address)
  t1/7 -> Accumulator_instance7/3(address)
  t1/8 -> Accumulator_instance8/3(address)
  t1/9 -> Accumulator_instance9/3(address)
  t1/10 -> Accumulator_instance10/3(address)
  t1/11 -> Accumulator_instance11/3(address)
  t1/12 -> Accumulator_instance12/3(address)
  t1/13 -> Accumulator_instance13/3(address)
  t1/14 -> Accumulator_instance14/3(address)
  t1/15 -> Accumulator_instance15/3(address)
  t1/16 -> Accumulator_instance16/3(address)
  t1/17 -> Accumulator_instance17/3(address)
  t1/18 -> Accumulator_instance18/3(address)
  t1/19 -> Accumulator_instance19/3(address)
  t1/20 -> Accumulator_instance20/3(address)
  t1/21 -> Accumulator_instance21/3(address)
  t1/22 -> Accumulator_instance22/3(address)
  t1/23 -> Accumulator_instance23/3(address)
  t1/24 -> Accumulator_instance24/3(address)
  t1/25 -> Accumulator_instance25/3(address)
  t1/26 -> Accumulator_instance26/3(address)
  t1/27 -> Accumulator_instance27/3(address)
  t1/28 -> Accumulator_instance28/3(address)
  t1/29 -> Accumulator_instance29/3(address)
  t1/30 -> Accumulator_instance30/3(address)
  t1/31 -> Accumulator_instance31/3(address)
  t1/32 -> Accumulator_instance32/3(address)
  t1/33 -> Accumulator_instance33/3(address)
  t1/34 -> Accumulator_instance34/3(address)
  t1/35 -> Accumulator_instance35/3(address)
  t1/36 -> Accumulator_instance36/3(address)
  t1/37 -> Accumulator_instance37/3(address)
  t1/38 -> Accumulator_instance38/3(address)
  t1/39 -> Accumulator_instance39/3(address)
  t1/40 -> Accumulator_instance40/3(address)
  t1/41 -> Accumulator_instance41/3(address)
  t1/42 -> Accumulator_instance42/3(address)
  t1/43 -> Accumulator_instance43/3(address)
  t1/44 -> Accumulator_instance44/3(address)
  t1/45 -> Accumulator_instance45/3(address)
  t1/46 -> Accumulator_instance46/3(address)
  t1/47 -> Accumulator_instance47/3(address)
  t1/48 -> Accumulator_instance48/3(address)
  t1/49 -> Accumulator_instance49/3(address)
  t1/50 -> Accumulator_instance50/3(address)
  t1/51 -> Accumulator_instance51/3(address)
  t1/52 -> Accumulator_instance52/3(address)
  t1/53 -> Accumulator_instance53/3(address)
  t1/54 -> Accumulator_instance54/3(address)
  t1/55 -> Accumulator_instance55/3(address)
  t1/56 -> Accumulator_instance56/3(address)
  t1/57 -> Accumulator_instance57/3(address)
  t1/58 -> Accumulator_instance58/3(address)
  t1/59 -> Accumulator_instance59/3(address)
  t1/60 -> Accumulator_instance60/3(address)
  t2/1 -> t3/1
  Accumulator_instance1/1(hps) -> t2/1
  Accumulator_instance2/1(hps) -> t2/2
  Accumulator_instance3/1(hps) -> t2/3
  Accumulator_instance4/1(hps) -> t2/4
  Accumulator_instance5/1(hps) -> t2/5
  Accumulator_instance6/1(hps) -> t2/6
  Accumulator_instance7/1(hps) -> t2/7
  Accumulator_instance8/1(hps) -> t2/8
  Accumulator_instance9/1(hps) -> t2/9
  Accumulator_instance10/1(hps) -> t2/10
  Accumulator_instance11/1(hps) -> t2/11
  Accumulator_instance12/1(hps) -> t2/12
  Accumulator_instance13/1(hps) -> t2/13
  Accumulator_instance14/1(hps) -> t2/14
  Accumulator_instance15/1(hps) -> t2/15
  Accumulator_instance16/1(hps) -> t2/16
  Accumulator_instance17/1(hps) -> t2/17
  Accumulator_instance18/1(hps) -> t2/18
  Accumulator_instance19/1(hps) -> t2/19
  Accumulator_instance20/1(hps) -> t2/20
  Accumulator_instance21/1(hps) -> t2/21
  Accumulator_instance22/1(hps) -> t2/22
  Accumulator_instance23/1(hps) -> t2/23
  Accumulator_instance24/1(hps) -> t2/24
  Accumulator_instance25/1(hps) -> t2/25
  Accumulator_instance26/1(hps) -> t2/26
  Accumulator_instance27/1(hps) -> t2/27
  Accumulator_instance28/1(hps) -> t2/28
  Accumulator_instance29/1(hps) -> t2/29
  Accumulator_instance30/1(hps) -> t2/30
  Accumulator_instance31/1(hps) -> t2/31
  Accumulator_instance32/1(hps) -> t2/32
  Accumulator_instance33/1(hps) -> t2/33
  Accumulator_instance34/1(hps) -> t2/34
  Accumulator_instance35/1(hps) -> t2/35
  Accumulator_instance36/1(hps) -> t2/36
  Accumulator_instance37/1(hps) -> t2/37
  Accumulator_instance38/1(hps) -> t2/38
  Accumulator_instance39/1(hps) -> t2/39
  Accumulator_instance40/1(hps) -> t2/40
  Accumulator_instance41/1(hps) -> t2/41
  Accumulator_instance42/1(hps) -> t2/42
  Accumulator_instance43/1(hps) -> t2/43
  Accumulator_instance44/1(hps) -> t2/44
  Accumulator_instance45/1(hps) -> t2/45
  Accumulator_instance46/1(hps) -> t2/46
  Accumulator_instance47/1(hps) -> t2/47
  Accumulator_instance48/1(hps) -> t2/48
  Accumulator_instance49/1(hps) -> t2/49
  Accumulator_instance50/1(hps) -> t2/50
  Accumulator_instance51/1(hps) -> t2/51
  Accumulator_instance52/1(hps) -> t2/52
  Accumulator_instance53/1(hps) -> t2/53
  Accumulator_instance54/1(hps) -> t2/54
  Accumulator_instance55/1(hps) -> t2/55
  Accumulator_instance56/1(hps) -> t2/56
  Accumulator_instance57/1(hps) -> t2/57
  Accumulator_instance58/1(hps) -> t2/58
  Accumulator_instance59/1(hps) -> t2/59
  Accumulator_instance60/1(hps) -> t2/60
  shift/1 -> t/1
  hough_address/1 -> Switch/1
  edge/1 -> Multiport Switch1/3
  mode/1 -> delayMatch120/1, delayMatch118/1, delayMatch116/1, delayMatch114/1, delayMatch112/1, delayMatch110/1, delayMatch108/1, delayMatch106/1, delayMatch104/1, delayMatch102/1, delayMatch100/1, delayMatch98/1, delayMatch96/1, delayMatch94/1, delayMatch92/1, delayMatch90/1, delayMatch88/1, delayMatch86/1, delayMatch84/1, delayMatch82/1, delayMatch80/1, delayMatch78/1, delayMatch76/1, delayMatch74/1, delayMatch72/1, delayMatch70/1, delayMatch68/1, delayMatch66/1, delayMatch64/1, delayMatch62/1, delayMatch60/1, delayMatch58/1, delayMatch56/1, delayMatch54/1, delayMatch52/1, delayMatch50/1, delayMatch48/1, delayMatch46/1, delayMatch44/1, delayMatch42/1, delayMatch40/1, delayMatch38/1, delayMatch36/1, delayMatch34/1, delayMatch32/1, delayMatch30/1, delayMatch28/1, delayMatch26/1, delayMatch24/1, delayMatch22/1, delayMatch20/1, delayMatch18/1, delayMatch16/1, delayMatch14/1, delayMatch12/1, delayMatch10/1, delayMatch8/1, delayMatch6/1, delayMatch4/1, delayMatch2/1, delayMatch/1, Multiport Switch1/1
  read_address/1 -> Data Type Conversion/1
  clear/1 -> Multiport Switch1/2
  theta_index/1 -> Delay/1
  delayMatch2/1 -> Accumulator_instance1/2(mode)
  Data Type Conversion/1 -> delayMatch1/1
  delayMatch4/1 -> Accumulator_instance2/2(mode)
  delayMatch5/1 -> Accumulator_instance2/4(edge)
  delayMatch6/1 -> Accumulator_instance3/2(mode)
  delayMatch7/1 -> Accumulator_instance3/4(edge)
  delayMatch8/1 -> Accumulator_instance4/2(mode)
  delayMatch9/1 -> Accumulator_instance4/4(edge)
  delayMatch10/1 -> Accumulator_instance5/2(mode)
  delayMatch11/1 -> Accumulator_instance5/4(edge)
  delayMatch12/1 -> Accumulator_instance6/2(mode)
  delayMatch13/1 -> Accumulator_instance6/4(edge)
  delayMatch14/1 -> Accumulator_instance7/2(mode)
  delayMatch15/1 -> Accumulator_instance7/4(edge)
  delayMatch16/1 -> Accumulator_instance8/2(mode)
  delayMatch17/1 -> Accumulator_instance8/4(edge)
  delayMatch18/1 -> Accumulator_instance9/2(mode)
  delayMatch19/1 -> Accumulator_instance9/4(edge)
  delayMatch20/1 -> Accumulator_instance10/2(mode)
  delayMatch21/1 -> Accumulator_instance10/4(edge)
  delayMatch22/1 -> Accumulator_instance11/2(mode)
  delayMatch23/1 -> Accumulator_instance11/4(edge)
  delayMatch24/1 -> Accumulator_instance12/2(mode)
  delayMatch25/1 -> Accumulator_instance12/4(edge)
  delayMatch26/1 -> Accumulator_instance13/2(mode)
  delayMatch27/1 -> Accumulator_instance13/4(edge)
  delayMatch28/1 -> Accumulator_instance14/2(mode)
  delayMatch29/1 -> Accumulator_instance14/4(edge)
  delayMatch30/1 -> Accumulator_instance15/2(mode)
  delayMatch31/1 -> Accumulator_instance15/4(edge)
  delayMatch32/1 -> Accumulator_instance16/2(mode)
  delayMatch33/1 -> Accumulator_instance16/4(edge)
  delayMatch34/1 -> Accumulator_instance17/2(mode)
  delayMatch35/1 -> Accumulator_instance17/4(edge)
  delayMatch36/1 -> Accumulator_instance18/2(mode)
  delayMatch37/1 -> Accumulator_instance18/4(edge)
  delayMatch38/1 -> Accumulator_instance19/2(mode)
  delayMatch39/1 -> Accumulator_instance19/4(edge)
  delayMatch40/1 -> Accumulator_instance20/2(mode)
  delayMatch41/1 -> Accumulator_instance20/4(edge)
  delayMatch42/1 -> Accumulator_instance21/2(mode)
  delayMatch43/1 -> Accumulator_instance21/4(edge)
  delayMatch44/1 -> Accumulator_instance22/2(mode)
  delayMatch45/1 -> Accumulator_instance22/4(edge)
  delayMatch46/1 -> Accumulator_instance23/2(mode)
  delayMatch47/1 -> Accumulator_instance23/4(edge)
  delayMatch48/1 -> Accumulator_instance24/2(mode)
  delayMatch49/1 -> Accumulator_instance24/4(edge)
  delayMatch50/1 -> Accumulator_instance25/2(mode)
  delayMatch51/1 -> Accumulator_instance25/4(edge)
  delayMatch52/1 -> Accumulator_instance26/2(mode)
  delayMatch53/1 -> Accumulator_instance26/4(edge)
  delayMatch54/1 -> Accumulator_instance27/2(mode)
  delayMatch55/1 -> Accumulator_instance27/4(edge)
  delayMatch56/1 -> Accumulator_instance28/2(mode)
  delayMatch57/1 -> Accumulator_instance28/4(edge)
  delayMatch58/1 -> Accumulator_instance29/2(mode)
  delayMatch59/1 -> Accumulator_instance29/4(edge)
  delayMatch60/1 -> Accumulator_instance30/2(mode)
  delayMatch61/1 -> Accumulator_instance30/4(edge)
  delayMatch62/1 -> Accumulator_instance31/2(mode)
  delayMatch63/1 -> Accumulator_instance31/4(edge)
  delayMatch64/1 -> Accumulator_instance32/2(mode)
  delayMatch65/1 -> Accumulator_instance32/4(edge)
  delayMatch66/1 -> Accumulator_instance33/2(mode)
  delayMatch67/1 -> Accumulator_instance33/4(edge)
  delayMatch68/1 -> Accumulator_instance34/2(mode)
  delayMatch69/1 -> Accumulator_instance34/4(edge)
  delayMatch70/1 -> Accumulator_instance35/2(mode)
  delayMatch71/1 -> Accumulator_instance35/4(edge)
  delayMatch72/1 -> Accumulator_instance36/2(mode)
  delayMatch73/1 -> Accumulator_instance36/4(edge)
  delayMatch74/1 -> Accumulator_instance37/2(mode)
  delayMatch75/1 -> Accumulator_instance37/4(edge)
  delayMatch76/1 -> Accumulator_instance38/2(mode)
  delayMatch77/1 -> Accumulator_instance38/4(edge)
  delayMatch78/1 -> Accumulator_instance39/2(mode)
  delayMatch79/1 -> Accumulator_instance39/4(edge)
  delayMatch80/1 -> Accumulator_instance40/2(mode)
  delayMatch81/1 -> Accumulator_instance40/4(edge)
  delayMatch82/1 -> Accumulator_instance41/2(mode)
  delayMatch83/1 -> Accumulator_instance41/4(edge)
  delayMatch84/1 -> Accumulator_instance42/2(mode)
  delayMatch85/1 -> Accumulator_instance42/4(edge)
  delayMatch86/1 -> Accumulator_instance43/2(mode)
  delayMatch87/1 -> Accumulator_instance43/4(edge)
  delayMatch88/1 -> Accumulator_instance44/2(mode)
  delayMatch89/1 -> Accumulator_instance44/4(edge)
  delayMatch90/1 -> Accumulator_instance45/2(mode)
  delayMatch91/1 -> Accumulator_instance45/4(edge)
  delayMatch92/1 -> Accumulator_instance46/2(mode)
  delayMatch93/1 -> Accumulator_instance46/4(edge)
  delayMatch94/1 -> Accumulator_instance47/2(mode)
  delayMatch95/1 -> Accumulator_instance47/4(edge)
  delayMatch96/1 -> Accumulator_instance48/2(mode)
  delayMatch97/1 -> Accumulator_instance48/4(edge)
  delayMatch98/1 -> Accumulator_instance49/2(mode)
  delayMatch99/1 -> Accumulator_instance49/4(edge)
  delayMatch100/1 -> Accumulator_instance50/2(mode)
  delayMatch101/1 -> Accumulator_instance50/4(edge)
  delayMatch102/1 -> Accumulator_instance51/2(mode)
  delayMatch103/1 -> Accumulator_instance51/4(edge)
  delayMatch104/1 -> Accumulator_instance52/2(mode)
  delayMatch105/1 -> Accumulator_instance52/4(edge)
  delayMatch106/1 -> Accumulator_instance53/2(mode)
  delayMatch107/1 -> Accumulator_instance53/4(edge)
  delayMatch108/1 -> Accumulator_instance54/2(mode)
  delayMatch109/1 -> Accumulator_instance54/4(edge)
  delayMatch110/1 -> Accumulator_instance55/2(mode)
  delayMatch111/1 -> Accumulator_instance55/4(edge)
  delayMatch112/1 -> Accumulator_instance56/2(mode)
  delayMatch113/1 -> Accumulator_instance56/4(edge)
  delayMatch114/1 -> Accumulator_instance57/2(mode)
  delayMatch115/1 -> Accumulator_instance57/4(edge)
  delayMatch116/1 -> Accumulator_instance58/2(mode)
  delayMatch117/1 -> Accumulator_instance58/4(edge)
  delayMatch118/1 -> Accumulator_instance59/2(mode)
  delayMatch119/1 -> Accumulator_instance59/4(edge)
  delayMatch120/1 -> Accumulator_instance60/2(mode)
  delayMatch121/1 -> Accumulator_instance60/4(edge)
  Multiport Switch1/1 -> delayMatch121/1, delayMatch119/1, delayMatch117/1, delayMatch115/1, delayMatch113/1, delayMatch111/1, delayMatch109/1, delayMatch107/1, delayMatch105/1, delayMatch103/1, delayMatch101/1, delayMatch99/1, delayMatch97/1, delayMatch95/1, delayMatch93/1, delayMatch91/1, delayMatch89/1, delayMatch87/1, delayMatch85/1, delayMatch83/1, delayMatch81/1, delayMatch79/1, delayMatch77/1, delayMatch75/1, delayMatch73/1, delayMatch71/1, delayMatch69/1, delayMatch67/1, delayMatch65/1, delayMatch63/1, delayMatch61/1, delayMatch59/1, delayMatch57/1, delayMatch55/1, delayMatch53/1, delayMatch51/1, delayMatch49/1, delayMatch47/1, delayMatch45/1, delayMatch43/1, delayMatch41/1, delayMatch39/1, delayMatch37/1, delayMatch35/1, delayMatch33/1, delayMatch31/1, delayMatch29/1, delayMatch27/1, delayMatch25/1, delayMatch23/1, delayMatch21/1, delayMatch19/1, delayMatch17/1, delayMatch15/1, delayMatch13/1, delayMatch11/1, delayMatch9/1, delayMatch7/1, delayMatch5/1, delayMatch3/1
  Delay/1 -> delayMatch122/1
